simulink model "wam_v_simulation"  (R2017b)
settings: Solver=VariableStepAuto  StartTime=0.0  StopTime=10.0  FixedStep=0.001  RelTol=1e-3
libraries: robotlib x8
settings Model: Creator=masaya  LastModifiedBy=masaya

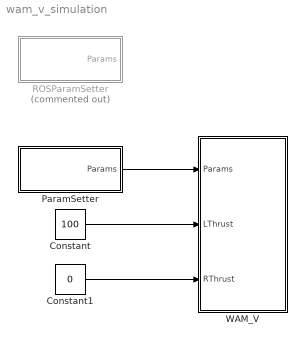
== system wam_v_simulation ==
  Constant : Constant  Value=100
  Constant1 : Constant  Value=0
  ParamSetter : Subsystem
  ROSParamSetter : Subsystem  Commented=on
  WAM_V : Subsystem
  wires:
  Constant/1 -> WAM_V/2(LThrust)
  Constant1/1 -> WAM_V/3(RThrust)
  ParamSetter/1(Params) -> WAM_V/1(Params)

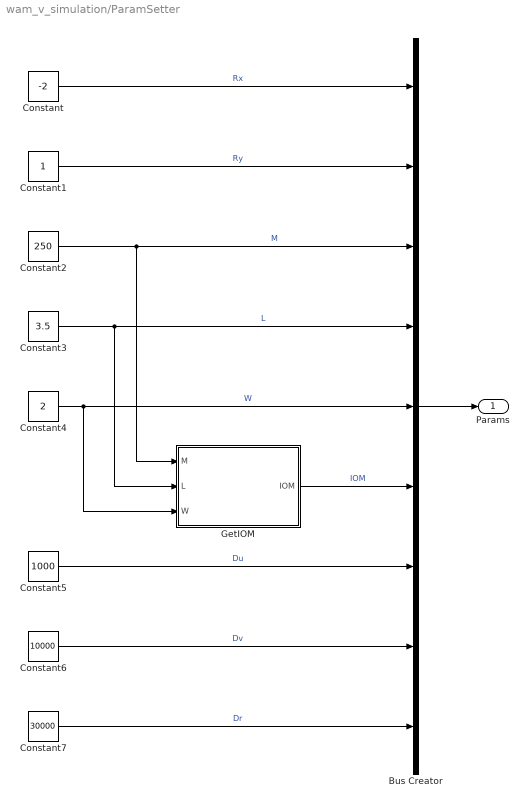
== system wam_v_simulation/ParamSetter ==
  Bus Creator : BusCreator  Inputs=9
  Constant : Constant  Value=-2
  Constant1 : Constant
  Constant2 : Constant  Value=250
  Constant3 : Constant  Value=3.5
  Constant4 : Constant  Value=2
  Constant5 : Constant  Value=1000
  Constant6 : Constant  Value=10000
  Constant7 : Constant  Value=30000
  GetIOM : Subsystem
  Params : Outport
  wires:
  Constant/1 -> Bus Creator/1  "Rx"
  Constant1/1 -> Bus Creator/2  "Ry"
  Constant2/1 -> GetIOM/1(M), Bus Creator/3  "M"
  Bus Creator/1 -> Params/1
  Constant3/1 -> GetIOM/2(L), Bus Creator/4  "L"
  Constant4/1 -> GetIOM/3(W), Bus Creator/5  "W"
  GetIOM/1(IOM) -> Bus Creator/6  "IOM"
  Constant5/1 -> Bus Creator/7  "Du"
  Constant6/1 -> Bus Creator/8  "Dv"
  Constant7/1 -> Bus Creator/9  "Dr"

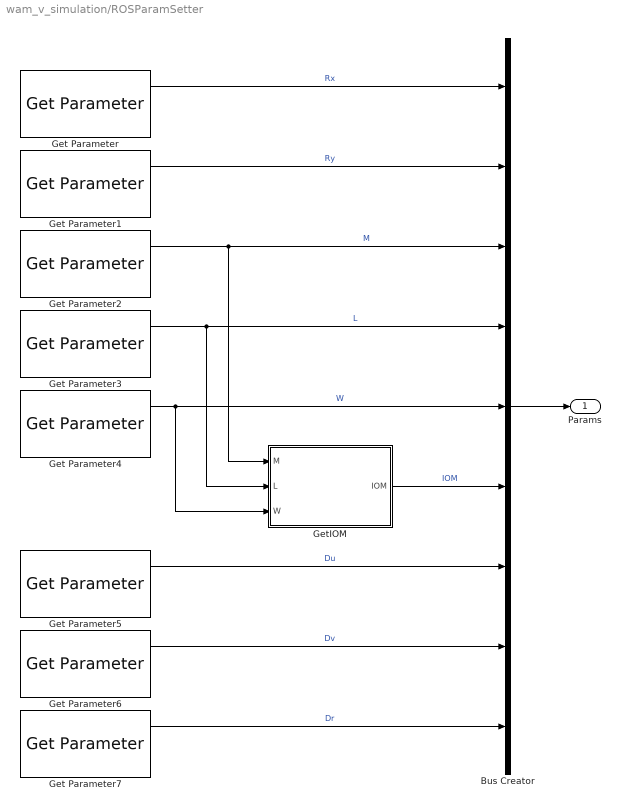
== system wam_v_simulation/ROSParamSetter ==
  Bus Creator : BusCreator  Inputs=9
  Get Parameter : robotlib/Get Parameter  SourceLibraryInfo=This block requires Robotics System Toolbox  ParameterSource=Specify your own  ParameterName=/wam_v_simulation/Rx  ParameterType=double  ParameterMaxArrayLength=16  ParameterInitialValue=-2  SampleTime=-1  ShowErrorCodeOutput=on  ModelName=wam_v_simulation  BlockId=ParamGet_wam_v_simulation_3
      settings: SourceProductName=Robotics System Toolbox  SourceProductBaseCode=RO
  Get Parameter1 : robotlib/Get Parameter  SourceLibraryInfo=This block requires Robotics System Toolbox  ParameterSource=Specify your own  ParameterName=/wam_v_simulation/Ry  ParameterType=double  ParameterMaxArrayLength=16  ParameterInitialValue=1.0  SampleTime=-1  ShowErrorCodeOutput=on  ModelName=wam_v_simulation  BlockId=ParamGet_wam_v_simulation_4
      settings: SourceProductName=Robotics System Toolbox  SourceProductBaseCode=RO
  Get Parameter2 : robotlib/Get Parameter  SourceLibraryInfo=This block requires Robotics System Toolbox  ParameterSource=Specify your own  ParameterName=/wam_v_simulation/M  ParameterType=double  ParameterMaxArrayLength=16  ParameterInitialValue=250  SampleTime=-1  ShowErrorCodeOutput=on  ModelName=wam_v_simulation  BlockId=ParamGet_wam_v_simulation_5
      settings: SourceProductName=Robotics System Toolbox  SourceProductBaseCode=RO
  Get Parameter3 : robotlib/Get Parameter  SourceLibraryInfo=This block requires Robotics System Toolbox  ParameterSource=Specify your own  ParameterName=/wam_v_simulation/L  ParameterType=double  ParameterMaxArrayLength=16  ParameterInitialValue=3.5  SampleTime=-1  ShowErrorCodeOutput=on  ModelName=wam_v_simulation  BlockId=ParamGet_wam_v_simulation_9
      settings: SourceProductName=Robotics System Toolbox  SourceProductBaseCode=RO
  Get Parameter4 : robotlib/Get Parameter  SourceLibraryInfo=This block requires Robotics System Toolbox  ParameterSource=Specify your own  ParameterName=/wam_v_simulation/W  ParameterType=double  ParameterMaxArrayLength=16  ParameterInitialValue=2  SampleTime=-1  ShowErrorCodeOutput=on  ModelName=wam_v_simulation  BlockId=ParamGet_wam_v_simulation_10
      settings: SourceProductName=Robotics System Toolbox  SourceProductBaseCode=RO
  Get Parameter5 : robotlib/Get Parameter  SourceLibraryInfo=This block requires Robotics System Toolbox  ParameterSource=Specify your own  ParameterName=/wam_v_simulation/Du  ParameterType=double  ParameterMaxArrayLength=16  ParameterInitialValue=1000  SampleTime=-1  ShowErrorCodeOutput=on  ModelName=wam_v_simulation  BlockId=ParamGet_wam_v_simulation_31
      settings: SourceProductName=Robotics System Toolbox  SourceProductBaseCode=RO
  Get Parameter6 : robotlib/Get Parameter  SourceLibraryInfo=This block requires Robotics System Toolbox  ParameterSource=Specify your own  ParameterName=/wam_v_simulation/Dv  ParameterType=double  ParameterMaxArrayLength=16  ParameterInitialValue=10000  SampleTime=-1  ShowErrorCodeOutput=on  ModelName=wam_v_simulation  BlockId=ParamGet_wam_v_simulation_32
      settings: SourceProductName=Robotics System Toolbox  SourceProductBaseCode=RO
  Get Parameter7 : robotlib/Get Parameter  SourceLibraryInfo=This block requires Robotics System Toolbox  ParameterSource=Specify your own  ParameterName=/wam_v_simulation/Dr  ParameterType=double  ParameterMaxArrayLength=16  ParameterInitialValue=30000  SampleTime=-1  ShowErrorCodeOutput=on  ModelName=wam_v_simulation  BlockId=ParamGet_wam_v_simulation_33
      settings: SourceProductName=Robotics System Toolbox  SourceProductBaseCode=RO
  GetIOM : Subsystem
  Params : Outport
  wires:
  Get Parameter/1 -> Bus Creator/1  "Rx"
  Get Parameter1/1 -> Bus Creator/2  "Ry"
  Get Parameter2/1 -> GetIOM/1(M), Bus Creator/3  "M"
  Bus Creator/1 -> Params/1
  Get Parameter3/1 -> GetIOM/2(L), Bus Creator/4  "L"
  Get Parameter4/1 -> GetIOM/3(W), Bus Creator/5  "W"
  GetIOM/1(IOM) -> Bus Creator/6  "IOM"
  Get Parameter5/1 -> Bus Creator/7  "Du"
  Get Parameter6/1 -> Bus Creator/8  "Dv"
  Get Parameter7/1 -> Bus Creator/9  "Dr"

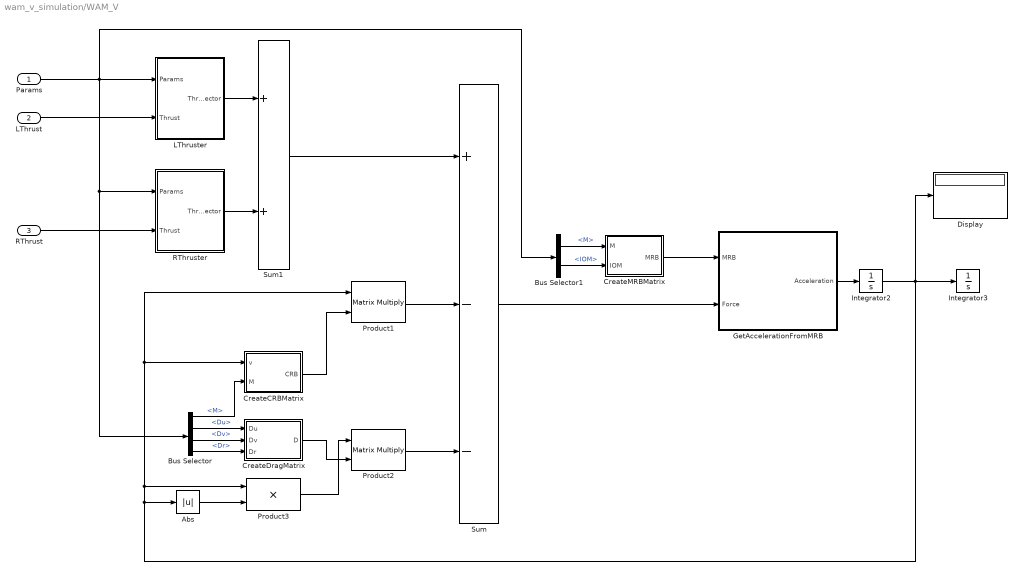
== system wam_v_simulation/WAM_V ==
  Params : Inport
  LThrust : Inport  Port=2
  RThrust : Inport  Port=3
  Abs : Abs
  Bus Selector : BusSelector  OutputSignals=M,Du,Dv,Dr
  Bus Selector1 : BusSelector  OutputSignals=M,IOM
  CreateCRBMatrix : MATLAB Function  TreatAsAtomicUnit=on
  CreateDragMatrix : MATLAB Function  TreatAsAtomicUnit=on
  CreateMRBMatrix : MATLAB Function  TreatAsAtomicUnit=on
  Display : Display
  GetAccelerationFromMRB : MATLAB Function  TreatAsAtomicUnit=on
  Integrator2 : Integrator
  Integrator3 : Integrator
  LThruster : Subsystem
  Product1 : Product  Multiplication=Matrix(*)
  Product2 : Product  Multiplication=Matrix(*)
  Product3 : Product
  RThruster : Subsystem
  Sum : Sum  Inputs=+--
  Sum1 : Sum
  wires:
  Params/1 -> Bus Selector1/1, Bus Selector/1, RThruster/1(Params), LThruster/1(Params)
  LThrust/1 -> LThruster/2(Thrust)
  RThrust/1 -> RThruster/2(Thrust)
  LThruster/1(ThrustVector) -> Sum1/1
  RThruster/1(ThrustVector) -> Sum1/2
  Bus Selector/2 -> CreateDragMatrix/1(Du)  "<Du>"
  Bus Selector/3 -> CreateDragMatrix/2(Dv)  "<Dv>"
  Bus Selector/4 -> CreateDragMatrix/3(Dr)  "<Dr>"
  Bus Selector/1 -> CreateCRBMatrix/2(M)  "<M>"
  Product2/1 -> Sum/3
  Integrator2/1 -> Display/1, Integrator3/1, CreateCRBMatrix/1(v), Product1/1, Product3/1, Abs/1
  Abs/1 -> Product3/2
  CreateCRBMatrix/1(CRB) -> Product1/2
  Product1/1 -> Sum/2
  Sum1/1 -> Sum/1
  CreateDragMatrix/1(D) -> Product2/2
  Product3/1 -> Product2/1
  Bus Selector1/1 -> CreateMRBMatrix/1(M)  "<M>"
  Bus Selector1/2 -> CreateMRBMatrix/2(IOM)  "<IOM>"
  CreateMRBMatrix/1(MRB) -> GetAccelerationFromMRB/1(MRB)
  Sum/1 -> GetAccelerationFromMRB/2(Force)
  GetAccelerationFromMRB/1(Acceleration) -> Integrator2/1

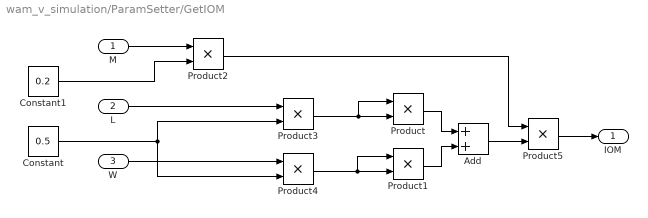
== system wam_v_simulation/ParamSetter/GetIOM ==
  M : Inport
  L : Inport  Port=2
  W : Inport  Port=3
  Add : Sum
  Constant : Constant  Value=0.5
  Constant1 : Constant  Value=0.2
  Product{,1..5} (6 alike) : Product
  IOM : Outport
  wires:
  Constant/1 -> Product4/2, Product3/2
  W/1 -> Product4/1
  L/1 -> Product3/1
  Product3/1 -> Product/2, Product/1
  Product4/1 -> Product1/1, Product1/2
  M/1 -> Product2/1
  Constant1/1 -> Product2/2
  Product/1 -> Add/1
  Product1/1 -> Add/2
  Add/1 -> Product5/2
  Product2/1 -> Product5/1
  Product5/1 -> IOM/1

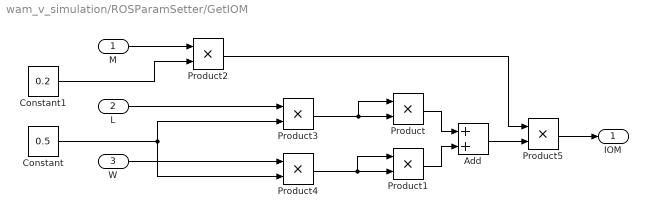
== system wam_v_simulation/ROSParamSetter/GetIOM ==
  M : Inport
  L : Inport  Port=2
  W : Inport  Port=3
  Add : Sum
  Constant : Constant  Value=0.5
  Constant1 : Constant  Value=0.2
  Product{,1..5} (6 alike) : Product
  IOM : Outport
  wires:
  Constant/1 -> Product4/2, Product3/2
  W/1 -> Product4/1
  L/1 -> Product3/1
  Product3/1 -> Product/2, Product/1
  Product4/1 -> Product1/1, Product1/2
  M/1 -> Product2/1
  Constant1/1 -> Product2/2
  Product/1 -> Add/1
  Product1/1 -> Add/2
  Add/1 -> Product5/2
  Product2/1 -> Product5/1
  Product5/1 -> IOM/1

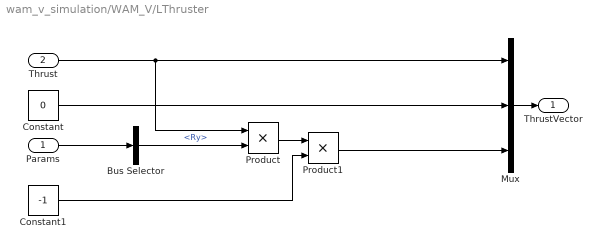
== system wam_v_simulation/WAM_V/LThruster ==
  Params : Inport
  Thrust : Inport  Port=2
  Bus Selector : BusSelector  OutputSignals=Ry
  Constant : Constant  Value=0
  Constant1 : Constant  Value=-1
  Mux : Mux  Inputs=3
  Product : Product
  Product1 : Product
  ThrustVector : Outport
  wires:
  Mux/1 -> ThrustVector/1
  Thrust/1 -> Product/1, Mux/1
  Constant/1 -> Mux/2
  Params/1 -> Bus Selector/1
  Bus Selector/1 -> Product/2  "<Ry>"
  Product/1 -> Product1/1
  Constant1/1 -> Product1/2
  Product1/1 -> Mux/3

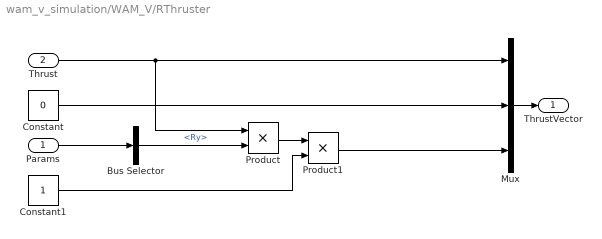
== system wam_v_simulation/WAM_V/RThruster ==
  Params : Inport
  Thrust : Inport  Port=2
  Bus Selector : BusSelector  OutputSignals=Ry
  Constant : Constant  Value=0
  Constant1 : Constant
  Mux : Mux  Inputs=3
  Product : Product
  Product1 : Product
  ThrustVector : Outport
  wires:
  Mux/1 -> ThrustVector/1
  Thrust/1 -> Product/1, Mux/1
  Constant/1 -> Mux/2
  Params/1 -> Bus Selector/1
  Bus Selector/1 -> Product/2  "<Ry>"
  Product/1 -> Product1/1
  Constant1/1 -> Product1/2
  Product1/1 -> Mux/3

== matlab function wam_v_simulation/WAM_V/CreateCRBMatrix ==
  data: v input; M input; CRB output
function CRB = fcn(v,M)

CRB=zeros(3,3);
CRB(1,2) = -M*v(2);
CRB(1,3) =  M*v(1);
CRB(2,1) =  M*v(2);
CRB(3,1) = -M*v(1);

== matlab function wam_v_simulation/WAM_V/CreateDragMatrix ==
  data: Du input; D output; Dv input; Dr input
function D = fcn(Du, Dv, Dr)

D = diag( [ Du, Dv, Dr ] );

== matlab function wam_v_simulation/WAM_V/CreateMRBMatrix ==
  data: M input; IOM input; MRB output
function MRB = fcn(M,IOM)

MRB=zeros(3,3);
MRB(1,1) = M;
MRB(2,2) = M;
MRB(3,3) = IOM;

== matlab function wam_v_simulation/WAM_V/GetAccelerationFromMRB ==
  data: MRB input; Force input; Acceleration output
function Acceleration = fcn(MRB,Force)
Acceleration = [0,0,0];
Acceleration(1) = Force(1)/MRB(1,1);
Acceleration(2) = Force(2)/MRB(2,2);
Acceleration(3) = Force(3)/MRB(3,3);
